simulink model "ControllerTesting"  (R2016a)
settings: Solver=VariableStepAuto  StartTime=0.0  StopTime=orbit_length*40  RelTol=1e-3
values from neighbouring files (symbols this model uses):
  A = eye(16,16)    [full_input_list.m]
  B = zeros(16,1)    [full_input_list.m]
  C = blkdiag(eye(3,3),zeros(3,3),eye(10,10))    [full_input_list.m]
  counter = 0    [full_input_list.m]
  deltaT = 0.00001    (= 1e-05)    [full_input_list.m]
  H = C    [full_input_list.m]
  kd = 0.5    [full_input_list.m]    (also in initACS.m = 0.01)
  kp = 1    [full_input_list.m]    (also in initACS.m = 0.01)
  OpModes = [0 0 0]    [full_input_list.m]
  OpTimes = [0 1 2]    [full_input_list.m]
  Q_k = zeros(16,16)    [full_input_list.m]
  R = R_k    [full_input_list.m]
  SeperationTime = 30000    [full_input_list.m]
  sim_start_time = (JD - JD_GPS0) * 24*60*60 - UTC_leap_seconds_wrt_GPS    (= 36000.0287935)    [full_input_list.m]
  st = 1/freq    (= 0.0125)    [full_input_list.m]    (also in initSimulink.m)
  u_k = zeros(16,1)    [full_input_list.m]
  w_k = zeros(16,1)    [full_input_list.m]
  x0 = [0 ... (first row only)    [full_input_list.m]
  Z_k = zeros(16,1)    [full_input_list.m]
undefined symbols (not defined in the file or in its folder): DiscIntNeverNeededParam, Earth, G_igrf, gyro_DCM_BS, H_igrf, I_undeployed, IAU, km, Kschmidt, mag_variance, n, R_mean, sat2, WGS84
libraries: simulink x29, dspmathops x21, aerolibtransform2 x21, aerolibutil x19, vrlib x14, aerolibgravity2 x5, dspinverses x4, SimMainLibrary x3, dspmtrx3 x1, lib_violet_env x1
(part 3 of 3)

== system ControllerTesting/Flight Computers/Center Cube Controller/Attitude Compensator/Not Deployed Modes (switch)/Detumbling Slew ==
  note: Regulator
      | - q_target = [0 0 0 1]
      | - w_target = [0 0 0]
  note: Markley Regulator
      | This regulator takes the current directional quaterion vector, the target quaterion, the intertial matrix, and the current angular velocity to determine the required torque necessary to the slew.
      |
      | The equation is 7.8 listed on page 290 of Fundamentals of Spacecraft Attitude Determination and Control. The input I is currently not defined. Also important to the equation is equation 7.2
  q_BN : Inport
  w_BN : Inport  Port=2
  "Inertia " : Inport  Port=3
  Action Port : ActionPort
  3x3 Cross Product : aerolibutil/3x3 Cross Product
  Add : Sum  Inputs=+++
  Gain : Gain  Gain=-1
  Gain1 : Gain  Gain=kp
  Gain2 : Gain  Gain=-1
  Gain3 : Gain  Gain=kd
  Gain4 : Gain  Gain=-1
  Product : Product  Multiplication=Matrix(*)
  Quaternion Inverse : aerolibutil/Quaternion Inverse
  Quaternion Multiplication : aerolibutil/Quaternion Multiplication
  Selector : Selector  InputPortWidth=4  IndexOptions=Index vector (dialog)  Indices=[1 2 3]  OutputSizes=1
  Target q : Constant  Value=[ 0 0 0 1 ]
  tau : Outport
  wires:
  q_BN/1 -> Quaternion Multiplication/1
  Quaternion Inverse/1 -> Quaternion Multiplication/2
  Target q/1 -> Quaternion Inverse/1
  Quaternion Multiplication/1 -> Selector/1
  Selector/1 -> Gain1/1
  Gain1/1 -> Gain/1
  Gain3/1 -> Gain2/1
  w_BN/1 -> 3x3 Cross Product/1, Gain3/1, Product/2
  Add/1 -> tau/1
  Gain/1 -> Add/1
  Gain2/1 -> Add/2
  "Inertia "/1 -> Product/1
  Product/1 -> 3x3 Cross Product/2
  3x3 Cross Product/1 -> Gain4/1
  Gain4/1 -> Add/3

== system ControllerTesting/Flight Computers/Center Cube Controller/Attitude Compensator/Not Deployed Modes (switch)/Inital Spin Up ==
  note: Regulator
      | - q_target = [0 0 0 1]
      | - w_target = [0 0 0]
  note: Markley Regulator
      | This regulator takes the current directional quaterion vector, the target quaterion, the intertial matrix, and the current angular velocity to determine the required torque necessary to the slew.
      |
      | The equation is 7.8 listed on page 290 of Fundamentals of Spacecraft Attitude Determination and Control. The input I is currently not defined. Also important to the equation is equation 7.2
  q_BN : Inport
  w : Inport  Port=2
  "I " : Inport  Port=3
  Action Port : ActionPort
  3x3 Cross Product : aerolibutil/3x3 Cross Product
  Add : Sum  Inputs=+++
  Gain : Gain  Gain=-1
  Gain1 : Gain  Gain=kp
  Gain2 : Gain  Gain=-1
  Gain3 : Gain  Gain=kd
  Gain4 : Gain  Gain=-1
  Product : Product  Multiplication=Matrix(*)
  Quaternion Inverse : aerolibutil/Quaternion Inverse
  Quaternion Multiplication : aerolibutil/Quaternion Multiplication
  Selector : Selector  InputPortWidth=4  IndexOptions=Index vector (dialog)  Indices=[1 2 3]  OutputSizes=1
  Target q : Constant  Value=[ 0 0 0 1 ]
  tau : Outport
  wires:
  q_BN/1 -> Quaternion Multiplication/1
  Quaternion Inverse/1 -> Quaternion Multiplication/2
  Target q/1 -> Quaternion Inverse/1
  Quaternion Multiplication/1 -> Selector/1
  Selector/1 -> Gain1/1
  Gain1/1 -> Gain/1
  Gain3/1 -> Gain2/1
  w/1 -> Product/2, 3x3 Cross Product/1, Gain3/1
  Add/1 -> tau/1
  Gain/1 -> Add/1
  Gain2/1 -> Add/2
  "I "/1 -> Product/1
  Product/1 -> 3x3 Cross Product/2
  3x3 Cross Product/1 -> Gain4/1
  Gain4/1 -> Add/3

== system ControllerTesting/Flight Computers/Center Cube Controller/Attitude Compensator/Not Deployed Modes (switch)/Null Case1 ==
  Action Port : ActionPort
  Constant : Constant  Value=[ 0 0 0 ]
  Out1 : Outport
  wires:
  Constant/1 -> Out1/1

== system ControllerTesting/Flight Computers/Center Cube Controller/Attitude Compensator/Not Deployed Modes (switch)/Seek EKF Convergence ==
  Action Port : ActionPort
  Constant : Constant  Value=[ 0 0 0 ]
  Out1 : Outport
  wires:
  Constant/1 -> Out1/1

== system ControllerTesting/Flight Computers/Center Cube Controller/Attitude Compensator/Not Deployed Modes (switch)/Sun Pointing ==
  note: Regulator
      | - q_target = [0 0 1 0]
      | - w_target = [0 0 0]
  q : Inport
  w_BN : Inport  Port=2
  Action Port : ActionPort
  Add : Sum
  Add1 : Sum  Inputs=+-
  Gain : Gain  Gain=-1
  Gain1 : Gain  Gain=kp
  Gain2 : Gain  Gain=-1
  Gain3 : Gain  Gain=kd
  Quaternion Inverse : aerolibutil/Quaternion Inverse
  Quaternion Multiplication : aerolibutil/Quaternion Multiplication
  Selector : Selector  InputPortWidth=4  IndexOptions=Index vector (dialog)  Indices=[1 2 3]  OutputSizes=1
  Target q : Constant  Value=[ 0 0 1 0 ]
  Target w : Constant  Value=[ 0 0 0 ]
  tau : Outport
  wires:
  q/1 -> Quaternion Multiplication/1
  Quaternion Inverse/1 -> Quaternion Multiplication/2
  Target q/1 -> Quaternion Inverse/1
  Quaternion Multiplication/1 -> Selector/1
  Selector/1 -> Gain1/1
  Gain1/1 -> Gain/1
  Gain3/1 -> Gain2/1
  w_BN/1 -> Add1/1
  Add/1 -> tau/1
  Gain/1 -> Add/1
  Gain2/1 -> Add/2
  Target w/1 -> Add1/2
  Add1/1 -> Gain3/1

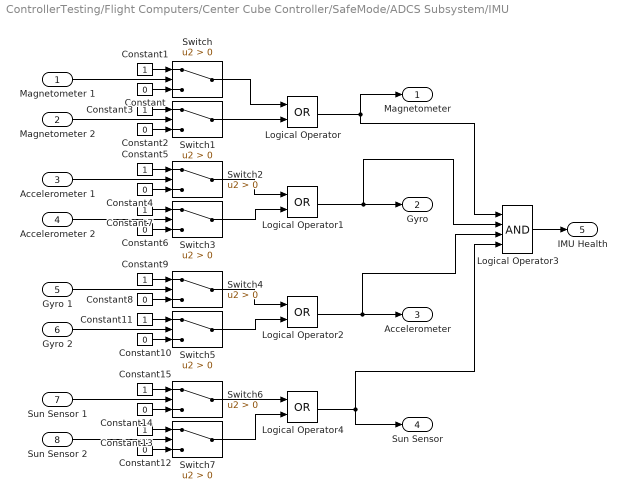
== system ControllerTesting/Flight Computers/Center Cube Controller/SafeMode/ADCS Subsystem/IMU ==
  Magnetometer 1 : Inport
  Magnetometer 2 : Inport  Port=2
  Accelerometer 1 : Inport  Port=3
  " Accelerometer 2" : Inport  Port=4
  Gyro 1 : Inport  Port=5
  Gyro 2 : Inport  Port=6
  Sun Sensor 1 : Inport  Port=7
  Sun Sensor 2 : Inport  Port=8
  Constant{,2,4,6,8,10,12,14} (8 alike) : Constant  Value=0
  Constant{1,3,5,7,9,11,13,15} (8 alike) : Constant
  Logical Operator{,1..2,4} (4 alike) : Logic  Operator=OR  AllPortsSameDT=off  OutDataTypeStr=boolean
  Logical Operator3 : Logic  Inputs=4  AllPortsSameDT=off  OutDataTypeStr=boolean
  Switch{,1..7} (8 alike) : Switch  Criteria=u2 > Threshold
  Magnetometer : Outport
  "Gyro " : Outport  Port=2
  Accelerometer : Outport  Port=3
  "Sun Sensor " : Outport  Port=4
  IMU Health : Outport  Port=5
  wires:
  Logical Operator3/1 -> IMU Health/1
  Switch7/1 -> Logical Operator4/2
  Constant12/1 -> Switch7/3
  Constant13/1 -> Switch7/1
  Switch6/1 -> Logical Operator4/1
  Constant14/1 -> Switch6/3
  Constant15/1 -> Switch6/1
  Logical Operator4/1 -> Logical Operator3/4, "Sun Sensor "/1
  Switch5/1 -> Logical Operator2/2
  Constant10/1 -> Switch5/3
  Constant11/1 -> Switch5/1
  Switch4/1 -> Logical Operator2/1
  Constant8/1 -> Switch4/3
  Constant9/1 -> Switch4/1
  Switch3/1 -> Logical Operator1/2
  Constant6/1 -> Switch3/3
  Constant7/1 -> Switch3/1
  Switch2/1 -> Logical Operator1/1
  Constant4/1 -> Switch2/3
  Constant5/1 -> Switch2/1
  Switch1/1 -> Logical Operator/2
  Constant2/1 -> Switch1/3
  Constant3/1 -> Switch1/1
  Switch/1 -> Logical Operator/1
  Constant/1 -> Switch/3
  Constant1/1 -> Switch/1
  Magnetometer 1/1 -> Switch/2
  Logical Operator2/1 -> Accelerometer/1, Logical Operator3/3
  Logical Operator1/1 -> "Gyro "/1, Logical Operator3/2
  Logical Operator/1 -> Logical Operator3/1, Magnetometer/1
  Magnetometer 2/1 -> Switch1/2
  Gyro 1/1 -> Switch4/2
  Gyro 2/1 -> Switch5/2
  Sun Sensor 1/1 -> Switch6/2
  Sun Sensor 2/1 -> Switch7/2
  " Accelerometer 2"/1 -> Switch3/2
  Accelerometer 1/1 -> Switch2/2

== system ControllerTesting/Flight Computers/Center Cube Controller/SafeMode/ADCS Subsystem/Magnetic Torquers ==
  Magnetorquer X1 : Inport
  Magnetometer Y1 : Inport  Port=2
  Magnetometer Z1 : Inport  Port=3
  Constant : Constant  Value=0
  Constant1 : Constant
  Constant4 : Constant  Value=0
  Constant5 : Constant
  Constant8 : Constant  Value=0
  Constant9 : Constant
  Logical Operator3 : Logic  Inputs=3  AllPortsSameDT=off  OutDataTypeStr=boolean
  Switch : Switch  Criteria=u2 > Threshold
  Switch2 : Switch  Criteria=u2 > Threshold
  Switch4 : Switch  Criteria=u2 > Threshold
  X Torquer Status : Outport
  "Y Torquer Status " : Outport  Port=2
  Z Torquer Status : Outport  Port=3
  Actuator Health : Outport  Port=4
  wires:
  Logical Operator3/1 -> Actuator Health/1
  Constant8/1 -> Switch4/3
  Constant9/1 -> Switch4/1
  Magnetometer Z1/1 -> Switch4/2
  Constant4/1 -> Switch2/3
  Constant5/1 -> Switch2/1
  Magnetometer Y1/1 -> Switch2/2
  Constant/1 -> Switch/3
  Constant1/1 -> Switch/1
  Magnetorquer X1/1 -> Switch/2
  Switch4/1 -> Z Torquer Status/1, Logical Operator3/3
  Switch2/1 -> "Y Torquer Status "/1, Logical Operator3/2
  Switch/1 -> X Torquer Status/1, Logical Operator3/1

== system ControllerTesting/Flight Computers/CenterCube EKF/x_measured/Lookup Tables/GPS time to Jd sfrom J2000 ==
  In1 : Inport
  Jd since GPS0 : Constant  Value=2444244.5
  Jd since J2000 : Constant  Value=2451545
  "Leap Seconds from GSP0 " : Constant  Value=27-9
  Sum : Sum  Inputs=|++
  Sum1 : Sum  Inputs=|++
  Sum2 : Sum  Inputs=|+-
  seconds to days conversion : Gain  Gain=1/86400
  Out1 : Outport
  wires:
  In1/1 -> Sum/1
  "Leap Seconds from GSP0 "/1 -> Sum/2
  Sum/1 -> seconds to days conversion/1
  seconds to days conversion/1 -> Sum1/1
  Jd since GPS0/1 -> Sum1/2
  Sum1/1 -> Sum2/1
  Jd since J2000/1 -> Sum2/2
  Sum2/1 -> Out1/1

== system ControllerTesting/Flight Computers/CenterCube EKF/x_measured/Lookup Tables/Sun position off of Jd frm J2000 ==
  In1 : Inport
  Gain : Gain  Gain=1.49597871e8
  MATLAB Function : MATLAB Function  TreatAsAtomicUnit=on
  Out1 : Outport
  wires:
  In1/1 -> MATLAB Function/1(J2000_days)
  MATLAB Function/1(S_ECI) -> Gain/1
  Gain/1 -> Out1/1

== system ControllerTesting/Flight Computers/CenterCube EKF/x_measured1/Lookup Tables/GPS time to Jd sfrom J2000 ==
  In1 : Inport
  Jd since GPS0 : Constant  Value=2444244.5
  Jd since J2000 : Constant  Value=2451545
  "Leap Seconds from GSP0 " : Constant  Value=27-9
  Sum : Sum  Inputs=|++
  Sum1 : Sum  Inputs=|++
  Sum2 : Sum  Inputs=|+-
  seconds to days conversion : Gain  Gain=1/86400
  Out1 : Outport
  wires:
  Sum2/1 -> Out1/1
  Jd since J2000/1 -> Sum2/2
  Sum1/1 -> Sum2/1
  Jd since GPS0/1 -> Sum1/2
  seconds to days conversion/1 -> Sum1/1
  Sum/1 -> seconds to days conversion/1
  "Leap Seconds from GSP0 "/1 -> Sum/2
  In1/1 -> Sum/1

== system ControllerTesting/Flight Computers/CenterCube EKF/x_measured1/Lookup Tables/Sun position off of Jd frm J2000 ==
  In1 : Inport
  Gain : Gain  Gain=1.49597871e8
  MATLAB Function : MATLAB Function  TreatAsAtomicUnit=on
  Out1 : Outport
  wires:
  Gain/1 -> Out1/1
  MATLAB Function/1(S_ECI) -> Gain/1
  In1/1 -> MATLAB Function/1(J2000_days)

== matlab function ControllerTesting/Flight Computers/CenterCube EKF/New State Prediction /A_LKF/MATLAB Function ==
  data: A input; A output; replacement input
function A = fcn(A,replacement)
%#codegen
A(13:16,10:12) = replacement;
end

== matlab function ControllerTesting/Inputs/Choose Mode ==
  data: time input; OM output; OpTimes input; OpModes input; SeperationTime input; SEPC output
function [OM , SEPC] = ...
    ModeSwitching(time,OpTimes,OpModes,SeperationTime)
%#codegen

tind = find(time > OpTimes);

if isempty(tind)
    i = 1;
else
    i = tind(end);
end

OM = OpModes(i);

if time > SeperationTime
    SEPC = 1;
else
    SEPC = 0;
end


end

== matlab function ControllerTesting/Flight Computers/Center Cube Controller/SafeMode/ACS State Machine Mode determination ==
  data: SafeMode_In input size=1; SafeMode_Out output; SafedOpMode output; PwbMEX output; t input; ADCSs input; EKFAE input size=13; EKFhs input; OpMode input; PbOpMode input size=1; SeperationCommand input
function [SafeMode_Out, SafedOpMode, PwbMEX] = fcn(SafeMode_In, ...
    t, ADCSs, EKFAE, EKFhs, OpMode, PbOpMode, SeperationCommand)
%#codegen
% x = t, ADCSs, EKFAE, EKFhs, OpMode, PbOpMode, SeperationCommand;
%% States of State Machine
% Time (From Deployment)​           t
% ADCS Health Status​               ADCSs
% EKF Attitude Estimate​            EKFAE
% EKF Health Status​                EKFhs
% Current Status                   OpMode
% PowerBoard Override              PbOpMode
% Deployed or not                  SeperationCommand

%% ADCSs
% ADCS Functional Status            ADCS_Fs
% ADCS Sectional Status             ADCS_Ss
% ADCS Component Status             ADCS_Cs

%%%%%%%%%%%%%%%%%%%%%%%%%%% MODE FLAGS %%%%%%%%%%%%%%%%%%%%%%%%%%%%%%%%%%%%
% 1 = Initial Charging Mode
% 2 = System Verification and Check Mode
% 3 = EPS THS Ping Mode
% 4 = FC THS Ping Mode
% 5 = Detumble Mode
% 6 = Sun Pointing Mode
% 7 = Spin Up Mode
% 8 = End Satellite Deployment Mode
% 9 = Normal OPS Mode
% 10 = Eclipse/Sleep Mode Mode
% 11 = Safe State Mode
% 12 = SeekingEKFConvergence

%% PwbMEX 
% PwbMEX is the error signal sent to the PowerBoard containing important
% information about the status of the ADCSs components as seen in safe
% mode. Informs that Safe Mode was entered, and requests an exit, as well
% as informs of the subsystem components that were not functionoing
% properly.
% MORE INFORMATION TO BE PROVIDED AFTER DISCUSSION WITH PADRAIG ON FORMAT
% AND NEED
SafedOpMode = 0;
SafeMode_Out = 0;
PwbMEX = zeros(1,8);
PwbMEX(1) = 0;
% Contact: Niccolo Porcari 2017

%%%%%%%%%%%%%%%%%%%%%%%%%%%%%%%%%%%%%%%%%%%%%%%%%%%%%%%%%%%%%%%%%%%%%%%%%%
    if t > 2700 % seconds
        % INITIAL CHECKS (check if in SafeMode)
        if (SafeMode_In == true || PbOpMode == 11)
            PwbMEX(1) = 1;
            % FIND A WAY TO INFORM POWERBOARD
            if (PbOpMode ~= 11)
                SafeMode_In = false;
                PwbMEX(1) = 0; % reset error message to powerboard
                OpMode = PbOpMode;
            else
                OpMode = 11;
                %% SAFE MODE OCCURS
                errorPositions = findADCSfault(ADCSs);
                % INFORM POWERBOARD Of location of error
                PwbMEX(2:8) = errorPositions; %%% PARTIAL ONLY
            end
        else
            %% SECTION for all modes where  ADCS is operational 
            % Pretend EKFhs is a boolean for now:
            if (OpMode == 5) || (OpMode == 6) || (OpMode == 7) || (OpMode == 9) || (OpMode == 10)
                if ADCSs(1) == false % Failure of ADCS trips Safe State Mode
                    OpMode = 11;
                    PwbMEX(1) = 1;
                    SafeMode_in = true;
                elseif EKFhs ~= true % Check validity of EKF estimate
                    OpMode = 12;  % Need to think of what we're gonna do if 
                                    % the EKF isn't technically accurate yet
                elseif EKFhs == true
                    OpMode = PbOpMode;
                end
            end
        end
        
        %% RESET OpMode to match PbOpMode 
        if (PbOpMode ~= OpMode && OpMode ~= 12) % set mode to match powerboard demand
            OpMode = PbOpMode;
        end
    end
end

== matlab function ControllerTesting/PowerBoard Simulation/Choose Mode ==
  data: PwbMEX input; time input; OM output; OpTimes input; OpModes input; SeperationTime input; SEPC output
function [OM , SEPC] = ...
    ModeSwitching(PwbMEX, time,OpTimes,OpModes,SeperationTime)
%#codegen

tind = find(time > OpTimes);

if isempty(tind)
    i = 1;
else
    i = tind(end);
end

OM = OpModes(i);

if time > SeperationTime
    SEPC = 1;
else
    SEPC = 0;
end


end

== matlab function ControllerTesting/Flight Computers/CenterCube EKF/x_measured/q_N from Sensors/quat From DCM ==
  data: Q input; q_N output; D output
function [q_N,D]  = fcn(Q)

    [V,D] = eig(Q);
    q_N = zeros(4,1);
    a = zeros(3,1);
    tol = 1e-10;
    
    if abs(real(D(1,1))-1) <= tol
        a(:,1) = real(V(:,1));
        phi = atan(abs(imag(D(2,2)))/real(D(2,2)));
    elseif abs(real(D(2,2))-1) <= tol
        a(:,1) = real(V(:,2));
        phi = atan(abs(imag(D(1,1)))/real(D(1,1)));
    elseif abs(real(D(3,3))-1) <= tol
        a(:,1) = real(V(:,3));
        phi = atan(abs(imag(D(1,1)))/real(D(1,1)));
    else 
        a(:,1) = [1;0;0];
        phi = 0;
    end
    
    q_N(1) = a(1)*sin(phi/2);
    q_N(2) = a(2)*sin(phi/2);
    q_N(3) = a(3)*sin(phi/2);
    q_N(4) = cos(phi/2);
end

== matlab function ControllerTesting/Flight Computers/Center Cube Controller/Torque Coil Management/Torque Coil Management/I_PWMOutput Function ==
  data: I_des input; pwm output size=[1 3]; unused input; dir output size=3
function [pwm, dir] = fcn(I_des,~)
% max voltage is 3.3V. limit in current is depedent on coil location:
% 0.8A for Iz, and 0.2A for Ix and Iy. An internal power computation has
% to be performed to ensure that the power consumption of the coils is no
% more than 3W.
    I_maxZ = 0.2;
    I_maxYX = 0.8;
    I_max = [I_maxYX; I_maxYX; I_maxZ]; % limits power output of the coils
                                        % for a total of 3W of power at
                                        % 3.3V
    if max(I_max) == I_maxYX
        I_max = I_max/2 + [0;0;I_maxZ/2];
    end
    I_magn = abs(I_des);    % outputs the unsigned magnitude of each I component
    dir = sign(I_des);      % outputs direction of current flow needed
    
    % No idea what what is going on here but the dimension don't work out
    % output needs to be a 1x3, not the 3x3 that's being outputed
    del_t = min(min(I_magn,  I_max))/I_max;
    pwm = del_t;
end

== matlab function ControllerTesting/Flight Computers/CenterCube EKF/New State Prediction /Predictions ==
  data: x_ko input; F output; x_kp output
function [F,x_kp] = fcn(x_ko)
%#codegen

% BASIC 
GM = 3.986e14;
%% EOMs:
% xdd = - GM*x/(x^2+y^2+z^2)^(3/2)
% ydd = - GM*y/(x^2+y^2+z^2)^(3/2)
% zdd = - GM*z/(x^2+y^2+z^2)^(3/2)
n = length(x_ko);
x = x_ko(1);
y = x_ko(2);
z = x_ko(3);

w1 = x_ko(n-6);
w2 = x_ko(n-5);
w3 = x_ko(n-4);
q1 = x_ko(n-3);
q2 = x_ko(n-2);
q3 = x_ko(n-1);
q4 = x_ko(n);

x_kp = zeros(n,1);
F = zeros(n,n);

%% predicted state estimate
x_kp(1) = x_ko(4);
x_kp(2) = x_ko(5);
x_kp(3) = x_ko(6);
x_kp(4) = -GM*x/(x^2+y^2+z^2)^(3/2); 
x_kp(5) = -GM*y/(x^2+y^2+z^2)^(3/2);
x_kp(6) = -GM*z/(x^2+y^2+z^2)^(3/2);

x_kp(n-3) = 0.5*(w1*q4-q3*w2+q2*w3);
x_kp(n-2) = 0.5*(w1*q3+q4*w2-q1*w3);
x_kp(n-1) = 0.5*(-w1*q2+q1*w2+q4*w3);
x_kp(n) = 0.5*(-w1*q1-q2*w2-q3*w3);

%% F matrix for predicted covariance estimate 
% F for x
F(1,4) = 1;
F(2,5) = 1;
F(3,6) = 1;
% F for xdot
F(4,4) = (3/2)*(2*x^2)/(x^2+y^2+z^2)^(5/2)-1/(x^2+y^2+z^2)^(3/2);
F(4,5) = (3/2)*2*x*y/(x^2+y^2+z^2)^(5/2);
F(4,6) = (3/2)*2*x*z/(x^2+y^2+z^2)^(5/2);

F(5,4) = (3/2)*2*x*y/(x^2+y^2+z^2)^(5/2);
F(5,5) = (3/2)*(2*y^2)/(x^2+y^2+z^2)^(5/2)-1/(x^2+y^2+z^2)^(3/2);
F(5,6) = (3/2)*2*y*z/(x^2+y^2+z^2)^(5/2);

F(6,4) = (3/2)*2*x*z/(x^2+y^2+z^2)^(5/2);
F(6,5) = (3/2)*2*y*z/(x^2+y^2+z^2)^(5/2);
F(6,6) = (3/2)*(2*z^2)/(x^2+y^2+z^2)^(5/2)-1/(x^2+y^2+z^2)^(3/2);

% F for xddot
% Leave as 0 to ensure no changes in thetadot
% 7-8-9

% F for thetadot
% Leave as 0 to ensure no changes in thetadot
% 10-11-12

% F for quaternion changes
F(n-3,n-6) = 0.5*q4;
F(n-3,n-5) = -0.5*q3;
F(n-3,n-4) = 0.5*q2;
F(n-3,n-3) = 0;
F(n-3,n-2) = 0.5*w3;
F(n-3,n-1) = -0.5*w2;
F(n-3,n) = 0.5*w1;

F(n-2,n-6) = 0.5*q3;
F(n-2,n-5) = 0.5*q4;
F(n-2,n-4) = -0.5*q1;
F(n-2,n-3) = -0.5*w3;
F(n-2,n-2) = 0;
F(n-2,n-1) = 0.5*w1;
F(n-2,n) = 0.5*w2;

F(n-1,n-6) = -0.5*q2;
F(n-1,n-5) = 0.5*q1;
F(n-1,n-4) = 0.5*q4;
F(n-1,n-3) = 0.5*w2;
F(n-1,n-2) = -0.5*w1;
F(n-1,n-1) = 0;
F(n-1,n) = 0.5*w3;

F(n,n-6) = -0.5*q1;
F(n,n-5) = -0.5*q2;
F(n,n-4) = -0.5*q3;
F(n,n-3) = -0.5*w1;
F(n,n-2) = -0.5*w2;
F(n,n-1) = -0.5*w3;
F(n,n) = 0;
end

== matlab function ControllerTesting/Flight Computers/CenterCube EKF/x_measured1/Lookup Tables/Sun position off of Jd frm J2000/MATLAB Function ==
  data: J2000_days input; S_ECI output
function S_ECI = sun_position(J2000_days)
% SUN_ECI  Calculate the cartesian coordinates of the sun (in AU)
%			  in the Earth Centered Inertial (ECI) reference frame
%			  with mean equator and equinox of J2000
%
% [S_ECI] = SUN_ECI(J2000_days)
%
% Arguments:
% J2000_days 	- UT Days elapsed since J2000 (1 January, 2000, 12 noon)
% S_ECI				- Sun vector in ECI, units of AU
%
% Todd Humphreys
% Author: Todd Humphreys
% Algorithm: Modified algorithm based on Astronomical Almanac 2001, pg C24
% Tested: Todd Humphreys, November 10, 2001
% 			 Within 0.01 degrees of ECI sun vector from Astronomical Almanac 


RAD = 57.29577951308232;

T   = (J2000_days)/36525;		% Julian centuries since J2000
L0  = (280.46645 + 36000.76983*T + 0.0003032*T^2)/RAD;	% Mean longitude of Sun
M   = (357.52910 + 35999.05030*T - 0.0001559*T^2 - 0.00000048*T^3)/RAD;	 % Mean anomaly
e   = 0.016708617 - 0.000042037*T - 0.0000001236*T^2;
C   = (1.914600 - 0.004817*T - 0.000014*T^2)*sin(M) + (0.019993 - 0.000101*T)*sin(2*M) + 0.000290*sin(3*M);
C   = C/RAD;
SL  = L0 + C;	% Ecliptic longitude
Ni  = M + C;	% Sun true Anomaly
R   = 1.000001018*(1-e^2)/(1+e*cos(Ni));  % Distance, Earth to Sun
SL = SL - (0.01397*T*100)/RAD;	% Correction to ecliptic longitude to reference to J200 equinox
Obl = (23.439291 - 0.0130042*T - 0.00000016*T^2 + 0.000000504*T^3)/RAD;	% Obliquity of ecliptic
SL     = (SL/(2*pi) - floor(SL/(2*pi)))*2*pi;	% Reduce to 2pi range
RA     = atan2(cos(Obl)*sin(SL),cos(SL));		% Right ascension	
Dec    = asin(sin(Obl).*sin(SL));				% Declination

S_ECI = [R*cos(SL); R*cos(Obl)*sin(SL); R*sin(Obl)*sin(SL)];

== matlab function ControllerTesting/Dynamics /Dynamics of the System ==
  data: x_ko input; Inertia input; torques input; xdot output
function xdot = fcn( x_ko, Inertia, torques)
%#codegen

% BASIC 
GM = 3.986e14;
%% EOMs:
% current design for x_ko
% x y z xdot ydot zdot  - - -  
% xdd = - GM*x/(x^2+y^2+z^2)^(3/2)
% ydd = - GM*y/(x^2+y^2+z^2)^(3/2)
% zdd = - GM*z/(x^2+y^2+z^2)^(3/2)
n = length(x_ko);
x = x_ko(1);
y = x_ko(2);
z = x_ko(3);

w1 = x_ko(n-6);
w2 = x_ko(n-5);
w3 = x_ko(n-4);
q1 = x_ko(n-3);
q2 = x_ko(n-2);
q3 = x_ko(n-1);
q4 = x_ko(n);

if ~(torques(1) == 0 && torques(2) == 0  && torques(3) == 0 )
    alpha = Inertia\torques;
else 
    alpha = [0;0;0];
end
x_kp = zeros(n,1);

%% predicted state estimate
x_kp(1) = x_ko(4);
x_kp(2) = x_ko(5);
x_kp(3) = x_ko(6);
x_kp(4) = -GM*x/(x^2+y^2+z^2)^(3/2); 
x_kp(5) = -GM*y/(x^2+y^2+z^2)^(3/2);
x_kp(6) = -GM*z/(x^2+y^2+z^2)^(3/2);
% rotation rate update
x_kp(n-6) = alpha(1);
x_kp(n-5) = alpha(2);
x_kp(n-4) = alpha(3);
% quaternion update
x_kp(n-3) = 0.5*(w1*q4-q3*w2+q2*w3);
x_kp(n-2) = 0.5*(w1*q3+q4*w2-q1*w3);
x_kp(n-1) = 0.5*(-w1*q2+q1*w2+q4*w3);
x_kp(n) = 0.5*(-w1*q1-q2*w2-q3*w3);

xdot=x_kp;
end

== matlab function ControllerTesting/Flight Computers/CenterCube EKF/x_measured/Lookup Tables/Sun position off of Jd frm J2000/MATLAB Function ==
  data: J2000_days input; S_ECI output
function S_ECI = sun_position(J2000_days)
% SUN_ECI  Calculate the cartesian coordinates of the sun (in AU)
%			  in the Earth Centered Inertial (ECI) reference frame
%			  with mean equator and equinox of J2000
%
% [S_ECI] = SUN_ECI(J2000_days)
%
% Arguments:
% J2000_days 	- UT Days elapsed since J2000 (1 January, 2000, 12 noon)
% S_ECI				- Sun vector in ECI, units of AU
%
% Todd Humphreys
% Author: Todd Humphreys
% Algorithm: Modified algorithm based on Astronomical Almanac 2001, pg C24
% Tested: Todd Humphreys, November 10, 2001
% 			 Within 0.01 degrees of ECI sun vector from Astronomical Almanac 


RAD = 57.29577951308232;

T   = (J2000_days)/36525;		% Julian centuries since J2000
L0  = (280.46645 + 36000.76983*T + 0.0003032*T^2)/RAD;	% Mean longitude of Sun
M   = (357.52910 + 35999.05030*T - 0.0001559*T^2 - 0.00000048*T^3)/RAD;	 % Mean anomaly
e   = 0.016708617 - 0.000042037*T - 0.0000001236*T^2;
C   = (1.914600 - 0.004817*T - 0.000014*T^2)*sin(M) + (0.019993 - 0.000101*T)*sin(2*M) + 0.000290*sin(3*M);
C   = C/RAD;
SL  = L0 + C;	% Ecliptic longitude
Ni  = M + C;	% Sun true Anomaly
R   = 1.000001018*(1-e^2)/(1+e*cos(Ni));  % Distance, Earth to Sun
SL = SL - (0.01397*T*100)/RAD;	% Correction to ecliptic longitude to reference to J200 equinox
Obl = (23.439291 - 0.0130042*T - 0.00000016*T^2 + 0.000000504*T^3)/RAD;	% Obliquity of ecliptic
SL     = (SL/(2*pi) - floor(SL/(2*pi)))*2*pi;	% Reduce to 2pi range
RA     = atan2(cos(Obl)*sin(SL),cos(SL));		% Right ascension	
Dec    = asin(sin(Obl).*sin(SL));				% Declination

S_ECI = [R*cos(SL); R*cos(Obl)*sin(SL); R*sin(Obl)*sin(SL)];

== matlab function ControllerTesting/Sensors BUSSED/Center Cube Sensors/Create Sun Vector/Sun position off of Jd frm J2000/MATLAB Function ==
  data: J2000_days input; S_ECI output
function S_ECI = sun_position(J2000_days)
% SUN_ECI  Calculate the cartesian coordinates of the sun (in AU)
%			  in the Earth Centered Inertial (ECI) reference frame
%			  with mean equator and equinox of J2000
%
% [S_ECI] = SUN_ECI(J2000_days)
%
% Arguments:
% J2000_days 	- UT Days elapsed since J2000 (1 January, 2000, 12 noon)
% S_ECI				- Sun vector in ECI, units of AU
%
% Todd Humphreys
% Author: Todd Humphreys
% Algorithm: Modified algorithm based on Astronomical Almanac 2001, pg C24
% Tested: Todd Humphreys, November 10, 2001
% 			 Within 0.01 degrees of ECI sun vector from Astronomical Almanac 


RAD = 57.29577951308232;

T   = (J2000_days)/36525;		% Julian centuries since J2000
L0  = (280.46645 + 36000.76983*T + 0.0003032*T^2)/RAD;	% Mean longitude of Sun
M   = (357.52910 + 35999.05030*T - 0.0001559*T^2 - 0.00000048*T^3)/RAD;	 % Mean anomaly
e   = 0.016708617 - 0.000042037*T - 0.0000001236*T^2;
C   = (1.914600 - 0.004817*T - 0.000014*T^2)*sin(M) + (0.019993 - 0.000101*T)*sin(2*M) + 0.000290*sin(3*M);
C   = C/RAD;
SL  = L0 + C;	% Ecliptic longitude
Ni  = M + C;	% Sun true Anomaly
R   = 1.000001018*(1-e^2)/(1+e*cos(Ni));  % Distance, Earth to Sun
SL = SL - (0.01397*T*100)/RAD;	% Correction to ecliptic longitude to reference to J200 equinox
Obl = (23.439291 - 0.0130042*T - 0.00000016*T^2 + 0.000000504*T^3)/RAD;	% Obliquity of ecliptic
SL     = (SL/(2*pi) - floor(SL/(2*pi)))*2*pi;	% Reduce to 2pi range
RA     = atan2(cos(Obl)*sin(SL),cos(SL));		% Right ascension	
Dec    = asin(sin(Obl).*sin(SL));				% Declination

S_ECI = [R*cos(SL); R*cos(Obl)*sin(SL); R*sin(Obl)*sin(SL)];

== matlab function ControllerTesting/Sensors BUSSED/Center Cube Sensors/Gyro/Bias ==
  data: w input; wn output; noise input
function wn = fcn(w, noise)
%#codegen
    
    % Add the bias to the rotation rate.
    wn = zeros(size(noise));
    for k = 1:size(noise, 2)
        wn(:, k) = w + noise(:, k);
    end
    
end

== matlab function ControllerTesting/Sensors MUXED/Center Cube Sensors/Create Sun Vector/Sun position off of Jd frm J2000/MATLAB Function ==
  data: J2000_days input; S_ECI output
function S_ECI = sun_position(J2000_days)
% SUN_ECI  Calculate the cartesian coordinates of the sun (in AU)
%			  in the Earth Centered Inertial (ECI) reference frame
%			  with mean equator and equinox of J2000
%
% [S_ECI] = SUN_ECI(J2000_days)
%
% Arguments:
% J2000_days 	- UT Days elapsed since J2000 (1 January, 2000, 12 noon)
% S_ECI				- Sun vector in ECI, units of AU
%
% Todd Humphreys
% Author: Todd Humphreys
% Algorithm: Modified algorithm based on Astronomical Almanac 2001, pg C24
% Tested: Todd Humphreys, November 10, 2001
% 			 Within 0.01 degrees of ECI sun vector from Astronomical Almanac 


RAD = 57.29577951308232;

T   = (J2000_days)/36525;		% Julian centuries since J2000
L0  = (280.46645 + 36000.76983*T + 0.0003032*T^2)/RAD;	% Mean longitude of Sun
M   = (357.52910 + 35999.05030*T - 0.0001559*T^2 - 0.00000048*T^3)/RAD;	 % Mean anomaly
e   = 0.016708617 - 0.000042037*T - 0.0000001236*T^2;
C   = (1.914600 - 0.004817*T - 0.000014*T^2)*sin(M) + (0.019993 - 0.000101*T)*sin(2*M) + 0.000290*sin(3*M);
C   = C/RAD;
SL  = L0 + C;	% Ecliptic longitude
Ni  = M + C;	% Sun true Anomaly
R   = 1.000001018*(1-e^2)/(1+e*cos(Ni));  % Distance, Earth to Sun
SL = SL - (0.01397*T*100)/RAD;	% Correction to ecliptic longitude to reference to J200 equinox
Obl = (23.439291 - 0.0130042*T - 0.00000016*T^2 + 0.000000504*T^3)/RAD;	% Obliquity of ecliptic
SL     = (SL/(2*pi) - floor(SL/(2*pi)))*2*pi;	% Reduce to 2pi range
RA     = atan2(cos(Obl)*sin(SL),cos(SL));		% Right ascension	
Dec    = asin(sin(Obl).*sin(SL));				% Declination

S_ECI = [R*cos(SL); R*cos(Obl)*sin(SL); R*sin(Obl)*sin(SL)];

== matlab function ControllerTesting/Sensors BUSSED/Center Cube Sensors/Create Sun Vector1/Sun position off of Jd frm J2000/MATLAB Function ==
  data: J2000_days input; S_ECI output
function S_ECI = sun_position(J2000_days)
% SUN_ECI  Calculate the cartesian coordinates of the sun (in AU)
%			  in the Earth Centered Inertial (ECI) reference frame
%			  with mean equator and equinox of J2000
%
% [S_ECI] = SUN_ECI(J2000_days)
%
% Arguments:
% J2000_days 	- UT Days elapsed since J2000 (1 January, 2000, 12 noon)
% S_ECI				- Sun vector in ECI, units of AU
%
% Todd Humphreys
% Author: Todd Humphreys
% Algorithm: Modified algorithm based on Astronomical Almanac 2001, pg C24
% Tested: Todd Humphreys, November 10, 2001
% 			 Within 0.01 degrees of ECI sun vector from Astronomical Almanac 


RAD = 57.29577951308232;

T   = (J2000_days)/36525;		% Julian centuries since J2000
L0  = (280.46645 + 36000.76983*T + 0.0003032*T^2)/RAD;	% Mean longitude of Sun
M   = (357.52910 + 35999.05030*T - 0.0001559*T^2 - 0.00000048*T^3)/RAD;	 % Mean anomaly
e   = 0.016708617 - 0.000042037*T - 0.0000001236*T^2;
C   = (1.914600 - 0.004817*T - 0.000014*T^2)*sin(M) + (0.019993 - 0.000101*T)*sin(2*M) + 0.000290*sin(3*M);
C   = C/RAD;
SL  = L0 + C;	% Ecliptic longitude
Ni  = M + C;	% Sun true Anomaly
R   = 1.000001018*(1-e^2)/(1+e*cos(Ni));  % Distance, Earth to Sun
SL = SL - (0.01397*T*100)/RAD;	% Correction to ecliptic longitude to reference to J200 equinox
Obl = (23.439291 - 0.0130042*T - 0.00000016*T^2 + 0.000000504*T^3)/RAD;	% Obliquity of ecliptic
SL     = (SL/(2*pi) - floor(SL/(2*pi)))*2*pi;	% Reduce to 2pi range
RA     = atan2(cos(Obl)*sin(SL),cos(SL));		% Right ascension	
Dec    = asin(sin(Obl).*sin(SL));				% Declination

S_ECI = [R*cos(SL); R*cos(Obl)*sin(SL); R*sin(Obl)*sin(SL)];

== matlab function ControllerTesting/Flight Computers/CenterCube EKF/x_measured1/q_N from Sensors/quat From DCM ==
  data: Q input; q_N output; D output
function [q_N,D]  = fcn(Q)

    [V,D] = eig(Q);
    q_N = zeros(4,1);
    a = zeros(3,1);
    tol = 1e-10;
    
    if abs(real(D(1,1))-1) <= tol
        a(:,1) = real(V(:,1));
        phi = atan(abs(imag(D(2,2)))/real(D(2,2)));
    elseif abs(real(D(2,2))-1) <= tol
        a(:,1) = real(V(:,2));
        phi = atan(abs(imag(D(1,1)))/real(D(1,1)));
    elseif abs(real(D(3,3))-1) <= tol
        a(:,1) = real(V(:,3));
        phi = atan(abs(imag(D(1,1)))/real(D(1,1)));
    else 
        a(:,1) = [1;0;0];
        phi = 0;
    end
    
    q_N(1) = a(1)*sin(phi/2);
    q_N(2) = a(2)*sin(phi/2);
    q_N(3) = a(3)*sin(phi/2);
    q_N(4) = cos(phi/2);
end

== matlab function ControllerTesting/Flight Computers/CenterCube EKF/x_measured1/Name change ==
  data: u input; y output
function y = fcn(u)
%#codegen

y = u;

== matlab function ControllerTesting/Flight Computers/CenterCube EKF/x_measured1/Name change1 ==
  data: u input; y output
function y = fcn(u)
%#codegen

y = u;

== matlab function ControllerTesting/Flight Computers/CenterCube EKF/x_measured1/vis viva ==
  data: x input; xdot output
function xdot = fcn(x)
%#codegen
GM = 3.986e14;
rotation_about_earth = [1;0;0]; % This is assumed for the orbit given by Cory
r = sqrt(x(1)^2+x(2)^2+x(3)^2);
v_mag = sqrt(GM/r);
xdot_cross = cross(rotation_about_earth, x);
xdot_hat = xdot_cross/norm(xdot_cross);
xdot = xdot_hat * v_mag;

== matlab function ControllerTesting/x_measured1/Lookup Tables/Sun position off of Jd frm J2000/MATLAB Function ==
  data: J2000_days input; S_ECI output
function S_ECI = sun_position(J2000_days)
% SUN_ECI  Calculate the cartesian coordinates of the sun (in AU)
%			  in the Earth Centered Inertial (ECI) reference frame
%			  with mean equator and equinox of J2000
%
% [S_ECI] = SUN_ECI(J2000_days)
%
% Arguments:
% J2000_days 	- UT Days elapsed since J2000 (1 January, 2000, 12 noon)
% S_ECI				- Sun vector in ECI, units of AU
%
% Todd Humphreys
% Author: Todd Humphreys
% Algorithm: Modified algorithm based on Astronomical Almanac 2001, pg C24
% Tested: Todd Humphreys, November 10, 2001
% 			 Within 0.01 degrees of ECI sun vector from Astronomical Almanac 


RAD = 57.29577951308232;

T   = (J2000_days)/36525;		% Julian centuries since J2000
L0  = (280.46645 + 36000.76983*T + 0.0003032*T^2)/RAD;	% Mean longitude of Sun
M   = (357.52910 + 35999.05030*T - 0.0001559*T^2 - 0.00000048*T^3)/RAD;	 % Mean anomaly
e   = 0.016708617 - 0.000042037*T - 0.0000001236*T^2;
C   = (1.914600 - 0.004817*T - 0.000014*T^2)*sin(M) + (0.019993 - 0.000101*T)*sin(2*M) + 0.000290*sin(3*M);
C   = C/RAD;
SL  = L0 + C;	% Ecliptic longitude
Ni  = M + C;	% Sun true Anomaly
R   = 1.000001018*(1-e^2)/(1+e*cos(Ni));  % Distance, Earth to Sun
SL = SL - (0.01397*T*100)/RAD;	% Correction to ecliptic longitude to reference to J200 equinox
Obl = (23.439291 - 0.0130042*T - 0.00000016*T^2 + 0.000000504*T^3)/RAD;	% Obliquity of ecliptic
SL     = (SL/(2*pi) - floor(SL/(2*pi)))*2*pi;	% Reduce to 2pi range
RA     = atan2(cos(Obl)*sin(SL),cos(SL));		% Right ascension	
Dec    = asin(sin(Obl).*sin(SL));				% Declination

S_ECI = [R*cos(SL); R*cos(Obl)*sin(SL); R*sin(Obl)*sin(SL)];

== matlab function ControllerTesting/x_measured1/Name change ==
  data: u input; y output
function y = fcn(u)
%#codegen

y = u;

== matlab function ControllerTesting/x_measured1/Name change1 ==
  data: u input; y output
function y = fcn(u)
%#codegen

y = u;

== matlab function ControllerTesting/x_measured1/q_N from Sensors/quat From DCM ==
  data: Q input; q_N output; D output
function [q_N,D]  = fcn(Q)

    [V,D] = eig(Q);
    q_N = zeros(4,1);
    a = zeros(3,1);
    tol = 1e-10;
    
    if abs(real(D(1,1))-1) <= tol
        a(:,1) = real(V(:,1));
        phi = atan(abs(imag(D(2,2)))/real(D(2,2)));
    elseif abs(real(D(2,2))-1) <= tol
        a(:,1) = real(V(:,2));
        phi = atan(abs(imag(D(1,1)))/real(D(1,1)));
    elseif abs(real(D(3,3))-1) <= tol
        a(:,1) = real(V(:,3));
        phi = atan(abs(imag(D(1,1)))/real(D(1,1)));
    else 
        a(:,1) = [1;0;0];
        phi = 0;
    end
    
    q_N(1) = a(1)*sin(phi/2);
    q_N(2) = a(2)*sin(phi/2);
    q_N(3) = a(3)*sin(phi/2);
    q_N(4) = cos(phi/2);
end

== matlab function ControllerTesting/x_measured1/vis viva ==
  data: x input; xdot output
function xdot = fcn(x)
%#codegen
GM = 3.986e14;
rotation_about_earth = [1;0;0]; % This is assumed for the orbit given by Cory
r = sqrt(x(1)^2+x(2)^2+x(3)^2);
v_mag = sqrt(GM/r);
xdot_cross = cross(rotation_about_earth, x);
xdot_hat = xdot_cross/norm(xdot_cross);
xdot = xdot_hat * v_mag;

== matlab function ControllerTesting/MATLAB Function ==
  data: u input; y output
function y = normalizeQuat(u)
%#codegen
y = [u(1:end-4); u(end-3:end)/norm(u(end-3:end))];
